simulink model "W_integ_SOA_demo_codegen"  (R2024b)
settings: Solver=FixedStepAuto  StartTime=0.0  StopTime=10.0  FixedStep=0.2  RelTol=1e-3
undefined symbols (not defined in the file or in its folder): call_a_f
settings Model: Tag=EP_AA_WRAPPER_INTEGRATION  Creator=nabilekhoury  LastModifiedBy=nabilekhoury
settings OptimizationCC: DefaultParameterBehavior=Inlined  EnhancedBackFolding=on  PassReuseOutputArgsAs=Individual arguments  ZeroExternalMemoryAtStartup=off  ZeroInternalMemoryAtStartup=off  OptimizeBlockOrder=speed  DifferentSizesBufferReuse=on  OptimizationCustomize=off  EfficientTunableParamExpr=on
settings DebuggingCC: ParameterTunabilityLossMsg=error
settings SFSimCC: MATLABDynamicMemAlloc=off  SimTargetLang=C++
settings RTWCC: Description=Embedded Coder  SystemTargetFile=ert.tlc  GenCodeOnly=on  TemplateMakefile=ert_default_tmf  CustomSourceCode="#include \"SOA_demo_codegen_adapter.h\""  CustomInitializer=sut_initialize();  TargetLang=C++  GPUComputeCapability=3.5
settings CodeAppCC: ForceParamTrailComments=on  IgnoreCustomStorageClasses=off  MaxIdLength=256  OperatorAnnotations=on  SimulinkDataObjDesc=on  SFDataObjDesc=on  CustomSymbolStrGlobalVar=w_$R$N$M  CustomSymbolStrType=w_$N$R$M_T  InsertBlockDesc=on
settings ERTTargetCC: TargetLangStandard=C++11 (ISO)  GenerateSampleERTMain=on  RootIOFormat=Structure reference  ERTCustomFileTemplate=example_file_process.tlc  DynamicArrayContainerType=coder::array

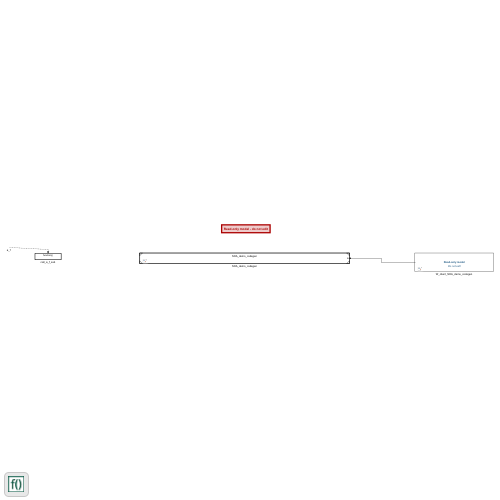
[thumbnail: Simulink's stored preview of the top-level diagram]
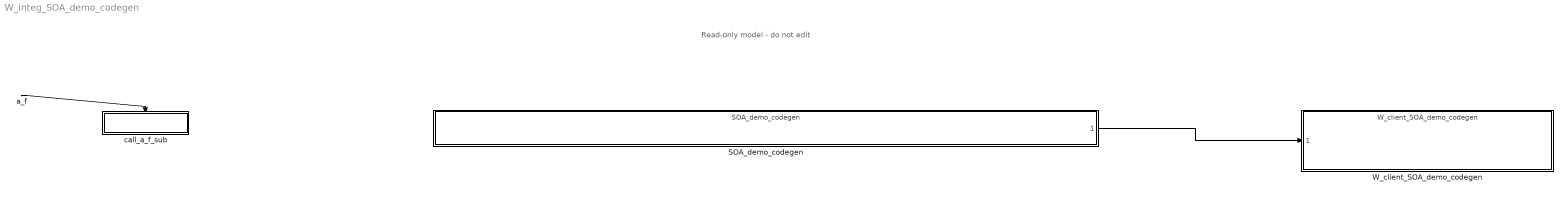
== system W_integ_SOA_demo_codegen ==
  note: Read-only model - do not edit
  a_f : Inport  OutputFunctionCall=on
  SOA_demo_codegen : ModelReference  Tag=BTC AUTOSAR Main Model Reference Block  ModelNameDialog=SOA_demo_codegen  SimulationMode=Normal  ScheduleRates=on  ModelReferenceVersion=1.4
  W_client_SOA_demo_codegen : ModelReference  ModelNameDialog=W_client_SOA_demo_codegen  SimulationMode=Normal  ScheduleRates=on  ModelReferenceVersion=1.1
      settings: OpenFcn=open_system(gcb, 'mask');
      mask DialogControl DescGroupVar Prompt: BTC Embedded Systems mocking block
      mask DialogControl DescTextVar Prompt: This is a BTC Embedded Systems mocking block. Do not edit its contents.
      mask Display: disp('\color[rgb]{0.11,0.34,0.51}\bf Read-only model', 'texmode', 'on');disp('\color[rgb]{0.11,0.34,0.51}\newline\newline\rm\it Do not edit', 'texmode', 'on');
  call_a_f_sub : Subsystem  TreatAsAtomicUnit=on
  wires:
  SOA_demo_codegen/1 -> W_client_SOA_demo_codegen/1
  a_f/1 -> call_a_f_sub/Trigger

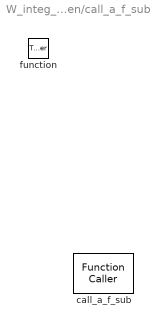
== system W_integ_SOA_demo_codegen/call_a_f_sub ==
  function : TriggerPort  TriggerType=function-call  VariantControl=(inherit)
  call_a_f_sub : FunctionCaller  FunctionPrototype=call_a_f()  InputArgumentSpecifications=<Enter example>  OutputArgumentSpecifications=<Enter example>
